simulink model "sd_filter_tb"  (R2022b)
settings: Solver=VariableStepAuto  StartTime=0.0  StopTime=t_stop  RelTol=1e-3
values from neighbouring files (symbols this model uses):
  ts = 1/fs    (= 8.85770975057e-08)    [check_example.m]    (also in sd_filter_top.m)
settings Model: Creator=Legion  LastModifiedBy=qaztr
settings SolverCC: AlgebraicLoopSolver=TrustRegion
settings DebuggingCC: UnconnectedInputMsg=warning  UnconnectedOutputMsg=warning  UnconnectedLineMsg=warning  SFMachineParentedDataDiag=warning
settings ModelReferenceCC: EnableRefExpFcnMdlSchedulingChecks=on
settings RTWCC: DLArmComputeVersion=19.05

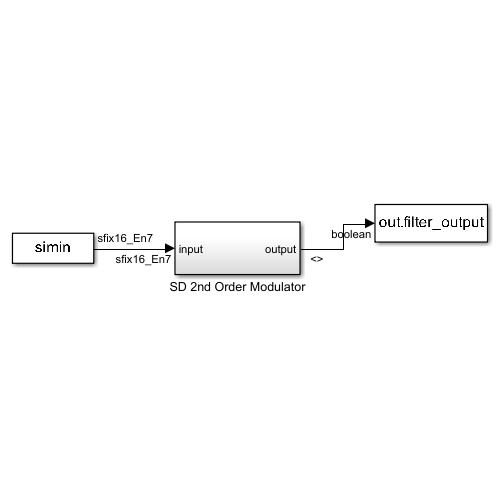
[thumbnail: Simulink's stored preview of the top-level diagram]
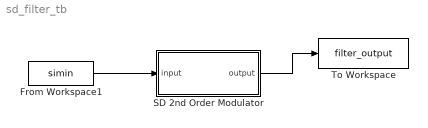
== system sd_filter_tb ==
  From Workspace1 : FromWorkspace  VariableName=simin  SampleTime=ts  Interpolate=off  OutputAfterFinalValue=Holding final value
  SD 2nd Order Modulator : Subsystem
  To Workspace : ToWorkspace  VariableName=filter_output  SaveFormat=Structure With Time  SampleTime=-1
  wires:
  SD 2nd Order Modulator/1(output) -> To Workspace/1
  From Workspace1/1 -> SD 2nd Order Modulator/1(input)

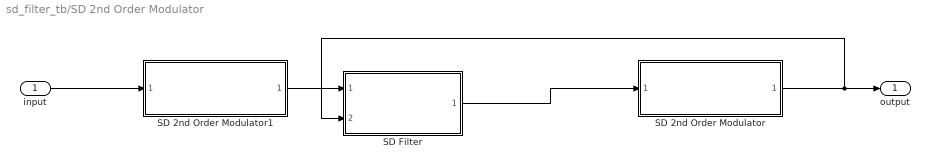
== system sd_filter_tb/SD 2nd Order Modulator ==
  input : Inport
  SD 2nd Order Modulator : Subsystem  ReferencedSubsystem=SD_2nd_Order_Modulator
  SD 2nd Order Modulator1 : Subsystem  ReferencedSubsystem=SD_2nd_Order_Modulator
  SD Filter : Subsystem  ReferencedSubsystem=SD_Filter
  output : Outport
  wires:
  SD Filter/1 -> SD 2nd Order Modulator/1
  SD 2nd Order Modulator/1 -> output/1, SD Filter/2
  SD 2nd Order Modulator1/1 -> SD Filter/1
  input/1 -> SD 2nd Order Modulator1/1
